simulink model "control_wrapper"  (R2020b)
settings: Solver=FixedStepDiscrete  StartTime=0.0  StopTime=10.0  RelTol=1e-3
settings Model: Creator=taste  LastModifiedBy=taste
settings DataIOCC: SaveOutput=off  SignalLogging=off  SaveTime=off
settings OptimizationCC: DefaultParameterBehavior=Inlined  UseDivisionForNetSlopeComputation=on  EnhancedBackFolding=on  PassReuseOutputArgsAs=Individual arguments  ZeroExternalMemoryAtStartup=off  ZeroInternalMemoryAtStartup=off  OptimizeBlockOrder=speed  DifferentSizesBufferReuse=on  OptimizationCustomize=off  EfficientTunableParamExpr=on
settings DebuggingCC: ParameterTunabilityLossMsg=error
settings SFSimCC: MATLABDynamicMemAlloc=off
settings RTWCC: Description=Embedded Coder  SystemTargetFile=ert.tlc  TemplateMakefile=ert_default_tmf  PostCodeGenCommand=packNGo(buildInfo);
settings CodeAppCC: ForceParamTrailComments=on  IgnoreCustomStorageClasses=off  OperatorAnnotations=on  SimulinkDataObjDesc=on  SFDataObjDesc=on  InsertBlockDesc=on
settings ERTTargetCC: TargetLangStandard=C99 (ISO)  GenerateSampleERTMain=on  InlinedParameterPlacement=NonHierarchical  ERTCustomFileTemplate=example_file_process.tlc

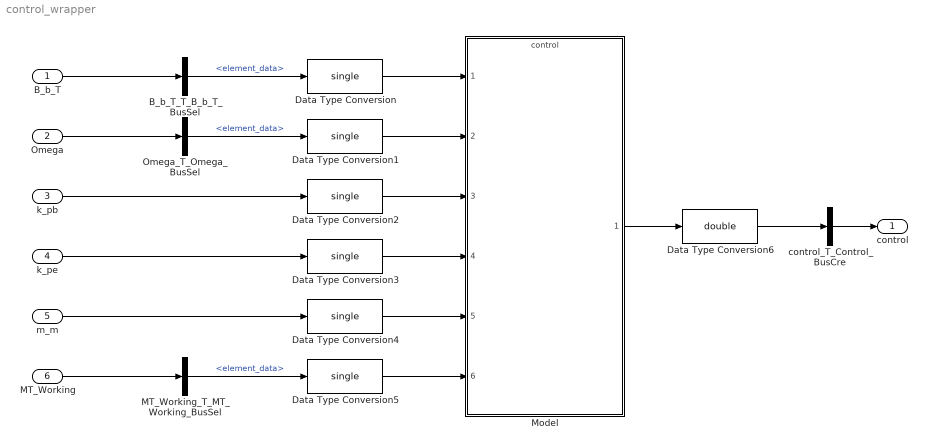
== system control_wrapper ==
  B_b_T : Inport  OutDataTypeStr=Bus: T_B_b_T  BusOutputAsStruct=on
  Omega : Inport  Port=2  OutDataTypeStr=Bus: T_Omega  BusOutputAsStruct=on
  k_pb : Inport  Port=3  OutDataTypeStr=T_Float  BusOutputAsStruct=on
  k_pe : Inport  Port=4  OutDataTypeStr=T_Float  BusOutputAsStruct=on
  m_m : Inport  Port=5  OutDataTypeStr=T_Float  BusOutputAsStruct=on
  MT_Working : Inport  Port=6  OutDataTypeStr=Bus: T_MT_Working  BusOutputAsStruct=on
  B_b_T_T_B_b_T_BusSel : BusSelector  OutputSignals=element_data
  Data Type Conversion{,1..5} (6 alike) : DataTypeConversion  OutDataTypeStr=single
  Data Type Conversion6 : DataTypeConversion  OutDataTypeStr=double
  MT_Working_T_MT_Working_BusSel : BusSelector  OutputSignals=element_data
  Model : ModelReference  ModelNameDialog=control.slx  SimulationMode=Normal  ModelReferenceVersion=5.5
  Omega_T_Omega_BusSel : BusSelector  OutputSignals=element_data
  control_T_Control_BusCre : BusCreator  Inputs=1  OutDataTypeStr=Bus: T_Control  NonVirtualBus=on
  control : Outport  OutDataTypeStr=Bus: T_Control  BusOutputAsStruct=on
  wires:
  Model/1 -> Data Type Conversion6/1
  Data Type Conversion/1 -> Model/1
  Data Type Conversion1/1 -> Model/2
  Data Type Conversion2/1 -> Model/3
  Data Type Conversion3/1 -> Model/4
  Data Type Conversion4/1 -> Model/5
  Data Type Conversion5/1 -> Model/6
  B_b_T/1 -> B_b_T_T_B_b_T_BusSel/1
  Omega/1 -> Omega_T_Omega_BusSel/1
  MT_Working/1 -> MT_Working_T_MT_Working_BusSel/1
  control_T_Control_BusCre/1 -> control/1
  B_b_T_T_B_b_T_BusSel/1 -> Data Type Conversion/1  "<element_data>"
  Omega_T_Omega_BusSel/1 -> Data Type Conversion1/1  "<element_data>"
  k_pb/1 -> Data Type Conversion2/1
  k_pe/1 -> Data Type Conversion3/1
  m_m/1 -> Data Type Conversion4/1
  MT_Working_T_MT_Working_BusSel/1 -> Data Type Conversion5/1  "<element_data>"
  Data Type Conversion6/1 -> control_T_Control_BusCre/1
